simulink model "hiv_model_ekf"  (R2021a)
settings: Solver=VariableStepAuto  StartTime=0.0  StopTime=100  RelTol=1e-3
values from neighbouring files (symbols this model uses):
  Delta = 0.01    [init.m]
  Theta = [0.25 50 0.25 10 0.01 0.0045]'    [init.m]
  xdash0 = [1000 550 0.0001]'    [init.m]
  xdash12RL = [1000 550]'    [init.m]
settings Model: Creator=schauer  LastModifiedBy=Tomo
settings SolverCC: AlgebraicLoopSolver=TrustRegion
settings DebuggingCC: SFMachineParentedDataDiag=warning

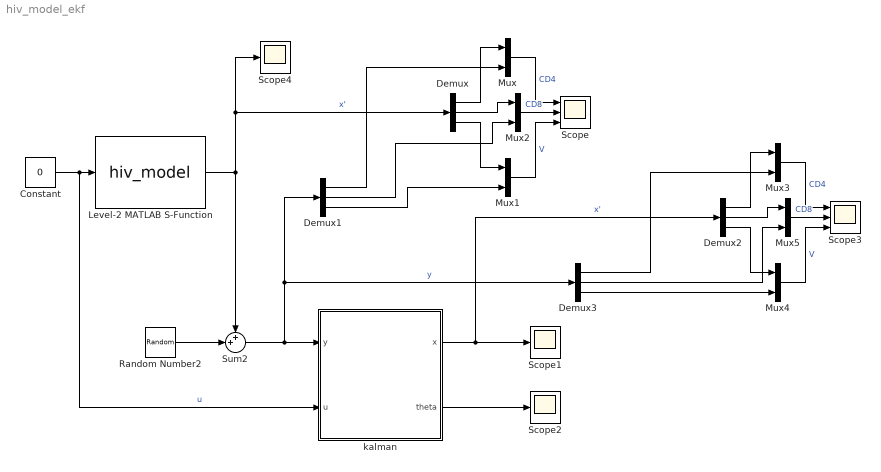
== system hiv_model_ekf ==
  Constant : Constant  Value=0
  Demux{,1..3} (4 alike) : Demux  Outputs=3
  Level-2 MATLAB S-Function : M-S-Function  FunctionName=hiv_model  Parameters=xdash0,Theta,xdash12RL
  Mux{,1..5} (6 alike) : Mux  Inputs=2
  Random Number2 : RandomNumber  Variance=[100 100 10^-5]  SampleTime=Delta
  Scope : Scope  NumInputPorts=3
  Scope1 : Scope
  Scope2 : Scope
  Scope3 : Scope  NumInputPorts=3
  Scope4 : Scope
  Sum2 : Sum  Inputs=++|
  kalman : MATLAB Function  TreatAsAtomicUnit=on
  wires:
  Constant/1 -> kalman/2(u), Level-2 MATLAB S-Function/1  "u"
  Level-2 MATLAB S-Function/1 -> Demux/1, Scope4/1, Sum2/1  "x'"
  Mux/1 -> Scope/1  "CD4"
  Demux/1 -> Mux/1
  Demux/3 -> Mux1/1
  Mux1/1 -> Scope/3  "V"
  Sum2/1 -> kalman/1(y), Demux3/1, Demux1/1  "y"
  Random Number2/1 -> Sum2/2
  Mux2/1 -> Scope/2  "CD8"
  Demux/2 -> Mux2/1
  Demux1/1 -> Mux/2
  Demux1/2 -> Mux2/2
  Demux1/3 -> Mux1/2
  kalman/2(theta) -> Scope2/1
  Demux3/1 -> Mux3/2
  Demux2/2 -> Mux5/1
  Mux5/1 -> Scope3/2  "CD8"
  Demux2/1 -> Mux3/1
  kalman/1(x) -> Scope1/1, Demux2/1  "x'"
  Mux3/1 -> Scope3/1  "CD4"
  Demux2/3 -> Mux4/1
  Demux3/3 -> Mux4/2
  Demux3/2 -> Mux5/2
  Mux4/1 -> Scope3/3  "V"

== matlab function hiv_model_ekf/kalman ==
  settings: updateMethod=DISCRETE
  data: y input; u input; x output; theta output
function [x, theta]  = fcn(y, u)

% init
persistent x_k P Z W
if isempty(x_k)
    
    % Kovarianzmatrix Z, W, P initializieren
    rng(0,'twister');
    v = [100 100 1e-5];
    x1_r = sqrt(v(1)).*randn(1000,1);
    x2_r = sqrt(v(2)).*randn(1000,1);
    x3_r = sqrt(v(3)).*randn(1000,1);
    Z = cov([x1_r, x2_r, x3_r]);
    W = 3^2 * eye(9);
%     W = 0 * eye(9)
    x_0 = [1000 550 0.0001]';
    th_wahr = [0.25 50 0.25 10 0.01 0.0045]';
    th_0 = th_wahr * (1 + 0.3);
    P = 0.3^2 * eye(9);
    
    x_k = zeros(1, 9);
    x_k(1:3) = x_0;
    x_k(4:9) = th_0;
end

Delta = 0.01;
x_RL = [1000 550]';

A_k = [(1-Delta*(x_k(4)-x_k(5)*x_k(3))),0,-Delta*x_k(4)*x_k(1),...
     Delta*(x_RL(1)-x_k(1)),Delta*x_k(1)*x_k(3),0,0,0,0;...                       
     0,(1-Delta*(x_k(6)+x_k(7)*x_k(3))),Delta*x_k(7)*x_k(2),0,0,...
     Delta*(x_RL(2)-x_k(2)),Delta*x_k(2)*x_k(3),0,0;...                           
     Delta*x_k(8)*x_k(3),-Delta*x_k(9)*x_k(3),1+Delta*(x_k(8)*x_k(1)-...
     x_k(9)*x_k(2)),0,0,0,0,Delta*x_k(1)*x_k(3),-Delta*x_k(2)*x_k(3);...    
     zeros(1,3),1,zeros(1,5);...                                            
     zeros(1,4),1,zeros(1,4);...                                            
     zeros(1,5),1,zeros(1,3);...                                            
     zeros(1,6),1,zeros(1,2);...                                            
     zeros(1,7),1,0;...                                                     
     zeros(1,8),1]; 

C = eye(3, 9);

% Prediktion
x_k = [x_k(1)+Delta*(x_k(4)*(x_RL(1)-x_k(1))-x_k(5)*x_k(1)*x_k(3)),...
      x_k(2)+Delta*(x_k(6)*(x_RL(2)-x_k(2))+x_k(7)*x_k(2)*x_k(3)),...
      x_k(3)+Delta*(x_k(3)*(x_k(8)*x_k(1)-x_k(9)*x_k(2))-u),...
      x_k(4:9)];
P = A_k*P*A_k' + W;

% Update
C_k1 = C;
K = P*C_k1' * (Z + C_k1*P*C_k1')^-1;
h_k = x_k(1:3);
x_k1 = x_k + (K*(y' - h_k)')';
P_k1 = P - K*C_k1*P;

% output
x = x_k1(1:3);
theta = x_k1(4:9);

x_k = x_k1;
P = P_k1;
